simulink model "clearing_faulted_segment_travelling_Wave"  (R2018a)
settings: Solver=ode23t  StartTime=0.0  StopTime=2  MaxStep=1e-3  RelTol=1e-3
values from neighbouring files (symbols this model uses):
  AC_lim = [1.5 -1.5]    [MT_HVDC_initialize.m]
  C_pm = 10.48e-3    (= 0.01048)    [MT_HVDC_initialize.m]
  ccsc_lim = [1.0 -1.0]    [MT_HVDC_initialize.m]
  DC_lim = [1.05 -1.05]    [MT_HVDC_initialize.m]
  f = 50    [MT_HVDC_initialize.m]
  Fc = 50    [MT_HVDC_initialize.m]
  Fn_filter = 1000    [MT_HVDC_initialize.m]
  Ireg_lim_i = [1.5, -1.5]    [MT_HVDC_initialize.m]
  Ireg_lim_r = [1.5, -1.5]    [MT_HVDC_initialize.m]
  Ki_ACreg_i = 260    [MT_HVDC_initialize.m]
  Ki_ccsc = 5    [MT_HVDC_initialize.m]
  Ki_DCreg_r = 150    [MT_HVDC_initialize.m]
  Ki_Ireg_i = 200    [MT_HVDC_initialize.m]
  Ki_Ireg_r = 100    [MT_HVDC_initialize.m]
  Ki_R_inv = 150000    [MT_HVDC_initialize.m]
  Ki_R_rec = 5000    [MT_HVDC_initialize.m]
  Kp_ACreg_i = 2    [MT_HVDC_initialize.m]
  Kp_ccsc = 1    [MT_HVDC_initialize.m]
  Kp_DCreg_r = 8    [MT_HVDC_initialize.m]
  Kp_Ireg_i = 2    [MT_HVDC_initialize.m]
  Kp_Ireg_r = 2    [MT_HVDC_initialize.m]
  Kp_R_inv = 0.001    [MT_HVDC_initialize.m]
  Kp_R_rec = 0.001    [MT_HVDC_initialize.m]
  L1_pu = 0.109    [MT_HVDC_initialize.m]
  L2_pu = 0.0824    [MT_HVDC_initialize.m]
  L_arm = L_arm_pu*Z_base66/w    [MT_HVDC_initialize.m]
  L_arm_pu = 0.15    [MT_HVDC_initialize.m]
  L_int = X_int/w    [MT_HVDC_initialize.m]
  n = 50    [MT_HVDC_initialize.m]
  n2 = 50    [MT_HVDC_initialize.m]
  P_nom = 220e6    (= 220000000)    [MT_HVDC_initialize.m]
  R1_pu = 0.00206    [MT_HVDC_initialize.m]
  R2_pu = 0.00206    [MT_HVDC_initialize.m]
  R_arm = 0.03    [MT_HVDC_initialize.m]
  R_arm_pu = R_arm/Z_base66    [MT_HVDC_initialize.m]
  R_int = sqrt((z_int_400^2)/(1+xr_ratio^2))    [MT_HVDC_initialize.m]
  Rg_T1 = 40    [MT_HVDC_initialize.m]
  S1_nom = P_nom    (= 220000000)    [MT_HVDC_initialize.m]
  S2_nom = P_nom    (= 220000000)    [MT_HVDC_initialize.m]
  T_fault = 1.4    [MT_HVDC_initialize.m]
  Ts_Control = 40e-6    (= 4e-05)    [MT_HVDC_initialize.m]
  Ts_Power = 20e-6    (= 2e-05)    [MT_HVDC_initialize.m]
  V1_prim = V_prim    (= 400000)    [MT_HVDC_initialize.m]
  V1_sec = V_grid    (= 66000)    [MT_HVDC_initialize.m]
  V2_prim = V_grid    (= 66000)    [MT_HVDC_initialize.m]
  V2_sec = 18e3    (= 18000)    [MT_HVDC_initialize.m]
  V_ac_ref = 1.035    [MT_HVDC_initialize.m]
  V_grid = 66e3    (= 66000)    [MT_HVDC_initialize.m]
  V_prim = 400e3    (= 400000)    [MT_HVDC_initialize.m]
  Vc_pm_r = 0*Vdc_nom/n    (= 0)    [MT_HVDC_initialize.m]
  Vdc_nom = 135e3    (= 135000)    [MT_HVDC_initialize.m]
  w = 2*pi*f    (= 314.159265359)    [MT_HVDC_initialize.m]
  z0z1 = 0.8    [MT_HVDC_initialize.m]
  Zeta_filter = 1    [MT_HVDC_initialize.m]
undefined symbols (not defined in the file or in its folder): D1, Delta, DiscIntNeverNeededParam
libraries: powerlib x417, powerlib_meascontrol x130, simulink x84, powerlib_extras x8, simulink_extras x5
(part 2 of 17)

== system clearing_faulted_segment_travelling_Wave/Extra Sequences and functionality (Normally turned off) ==
  note: Iq controllers for converters
  note: Used for start-up simulation
  Enable Harmonic Filters : Step  Time=0  SampleTime=0
  Enable Reactive power setpoint regulation - (iq reference for inverter) : Step  Time=0.1  SampleTime=0
  Energize Converters with startup current - Bypasses startup resistors : Step  Time=0  SampleTime=0
  Energize grid Harmonic Filter : Step  Time=0.1  SampleTime=0
  Grid Voltage stabilizer TURN ON - (iq reference for rectifier) : Step  Time=999  SampleTime=0
  tag scope: T_Energize=global, T_Harmonic1=global, T_iq_reg_i=global, T_iq_reg_r=global, T_startup=global
  wires:
  Energize grid Harmonic Filter/1 -> [T_Energize]
  Enable Reactive power setpoint regulation - (iq reference for inverter)/1 -> [T_iq_reg_i]
  Energize Converters with startup current - Bypasses startup resistors/1 -> [T_startup]
  Grid Voltage stabilizer TURN ON - (iq reference for rectifier)/1 -> [T_iq_reg_r]
  Enable Harmonic Filters/1 -> [T_Harmonic1]

== system clearing_faulted_segment_travelling_Wave/GENERATOR 1 ==
  C1 : powerlib/Measurements/Three-Phase V-I Measurement  VoltageMeasurement=phase-to-ground  SetLabelV=on  LabelV=VC1  Vpu=off  VpuLL=off  CurrentMeasurement=yes  SetLabelI=on  LabelI=IC1  Ipu=off  Pbase=100e6  Vbase=500e3  OutputType=Complex  PhasorSimulation=off  PSBequivalent=0
      settings: SourceProductName=Simscape Electrical
  Grid Equivalent1 : powerlib/Elements/Three-Phase Mutual Inductance Z1-Z0  LConnTagsString=a|b|c  RConnTagsString=A|B|C  PositiveSequence="[ R  L]"  ZeroSequence="[ z0z1*L*w/7  z0z1*L]*0"
      settings: SourceProductName=Simscape Electrical  SourceProductBaseCode=PS
  Internal Source Impedance2 : powerlib/Elements/Three-Phase Series RLC Branch  Commented=on  LConnTagsString=A|B|C  RConnTagsString=A|B|C  BranchType=RL  Resistance=R  Inductance=L  Capacitance=1e-6  Measurements=None
      settings: SourceProductName=Simscape Electrical
  Phase A - Programmable : powerlib/Electrical Sources/Three-Phase Programmable Voltage Source  PositiveSequence="[V_g  0 F_s]"  VariationEntity=Amplitude  VariationType=Table of time-amplitude pairs  VariationTypeAlt=Step  VariationStep=-0.5  VariationRate=10  VariationMagnitude=0.3  VariationFrequency=2  VariationTiming=[6 6.15]  VariationPhaseA=off  Amplitudes=[1 (1+A) 1]  TimeValues=[0 T1 (T1+T2)]  HarmonicGeneration=off  HarmonicA=[3 0.2 -25 0]  HarmonicB=[2 0.15 35 2]  Timing="[0.05  3]"  BusType=swing  Pref=0  Qref=0  Qmin=-inf  Qmax=inf
      settings: SourceProductName=Simscape Electrical
  Phase B,C - Programmable : powerlib/Electrical Sources/Three-Phase Programmable Voltage Source  PositiveSequence="[V_g  0 f]"  VariationEntity=Amplitude  VariationType=Table of time-amplitude pairs  VariationTypeAlt=Step  VariationStep=-0.5  VariationRate=10  VariationMagnitude=0.3  VariationFrequency=2  VariationTiming=[6 6.15]  VariationPhaseA=off  Amplitudes=[1 (1+BC) 1]  TimeValues=[0 T1 (T1+T2)]  HarmonicGeneration=off  HarmonicA=[3 0.2 -25 0]  HarmonicB=[2 0.15 35 2]  Timing="[0.05  3]"  BusType=swing  Pref=50e6  Qref=50e6  Qmin=-inf  Qmax=inf
      settings: SourceProductName=Simscape Electrical
  A : PMIOPort  Side=Right
  B : PMIOPort  Port=2  Side=Right
  C : PMIOPort  Port=3  Side=Right
  N : PMIOPort  Tag=PMCPort  Port=4  Side=Left
  connections:
  Phase B,C - Programmable/LConn1 -- Phase A - Programmable/LConn1 -- N/RConn1
  Grid Equivalent1/LConn1 -- Phase A - Programmable/RConn1
  Grid Equivalent1/LConn2 -- Phase B,C - Programmable/RConn2
  Grid Equivalent1/LConn3 -- Phase B,C - Programmable/RConn3
  Grid Equivalent1/RConn3 -- C1/LConn3
  Grid Equivalent1/RConn2 -- C1/LConn2
  Grid Equivalent1/RConn1 -- C1/LConn1
  C1/RConn1 -- A/RConn1
  C1/RConn2 -- B/RConn1
  C1/RConn3 -- C/RConn1

== system clearing_faulted_segment_travelling_Wave/GENERATOR 2 ==
  C2 : powerlib/Measurements/Three-Phase V-I Measurement  VoltageMeasurement=phase-to-ground  SetLabelV=on  LabelV=VC2  Vpu=off  VpuLL=off  CurrentMeasurement=yes  SetLabelI=on  LabelI=IC2  Ipu=off  Pbase=100e6  Vbase=500e3  OutputType=Complex  PhasorSimulation=off  PSBequivalent=0
      settings: SourceProductName=Simscape Electrical
  Grid Equivalent1 : powerlib/Elements/Three-Phase Mutual Inductance Z1-Z0  LConnTagsString=a|b|c  RConnTagsString=A|B|C  PositiveSequence="[ R  L]"  ZeroSequence="[ z0z1*L*w/7  z0z1*L]*0"
      settings: SourceProductName=Simscape Electrical  SourceProductBaseCode=PS
  Internal Source Impedance2 : powerlib/Elements/Three-Phase Series RLC Branch  Commented=on  LConnTagsString=A|B|C  RConnTagsString=A|B|C  BranchType=RL  Resistance=R  Inductance=L  Capacitance=1e-6  Measurements=None
      settings: SourceProductName=Simscape Electrical
  Phase A - Programmable : powerlib/Electrical Sources/Three-Phase Programmable Voltage Source  PositiveSequence="[V_g  0 F_s]"  VariationEntity=Amplitude  VariationType=Table of time-amplitude pairs  VariationTypeAlt=Step  VariationStep=-0.5  VariationRate=10  VariationMagnitude=0.3  VariationFrequency=2  VariationTiming=[6 6.15]  VariationPhaseA=off  Amplitudes=[1 (1+A) 1]  TimeValues=[0 T1 (T1+T2)]  HarmonicGeneration=off  HarmonicA=[3 0.2 -25 0]  HarmonicB=[2 0.15 35 2]  Timing="[0.05  3]"  BusType=swing  Pref=0  Qref=0  Qmin=-inf  Qmax=inf
      settings: SourceProductName=Simscape Electrical
  Phase B,C - Programmable : powerlib/Electrical Sources/Three-Phase Programmable Voltage Source  PositiveSequence="[V_g  0 f]"  VariationEntity=Amplitude  VariationType=Table of time-amplitude pairs  VariationTypeAlt=Step  VariationStep=-0.5  VariationRate=10  VariationMagnitude=0.3  VariationFrequency=2  VariationTiming=[6 6.15]  VariationPhaseA=off  Amplitudes=[1 (1+BC) 1]  TimeValues=[0 T1 (T1+T2)]  HarmonicGeneration=off  HarmonicA=[3 0.2 -25 0]  HarmonicB=[2 0.15 35 2]  Timing="[0.05  3]"  BusType=swing  Pref=50e6  Qref=50e6  Qmin=-inf  Qmax=inf
      settings: SourceProductName=Simscape Electrical
  A : PMIOPort  Side=Right
  B : PMIOPort  Port=2  Side=Right
  C : PMIOPort  Port=3  Side=Right
  N : PMIOPort  Tag=PMCPort  Port=4  Side=Left
  connections:
  Phase B,C - Programmable/LConn1 -- Phase A - Programmable/LConn1 -- N/RConn1
  Grid Equivalent1/LConn1 -- Phase A - Programmable/RConn1
  Grid Equivalent1/LConn2 -- Phase B,C - Programmable/RConn2
  Grid Equivalent1/LConn3 -- Phase B,C - Programmable/RConn3
  Grid Equivalent1/RConn3 -- C2/LConn3
  Grid Equivalent1/RConn2 -- C2/LConn2
  Grid Equivalent1/RConn1 -- C2/LConn1
  C2/RConn1 -- A/RConn1
  C2/RConn2 -- B/RConn1
  C2/RConn3 -- C/RConn1

== system clearing_faulted_segment_travelling_Wave/GENERATOR 3 ==
  C3 : powerlib/Measurements/Three-Phase V-I Measurement  VoltageMeasurement=phase-to-ground  SetLabelV=on  LabelV=VC3  Vpu=off  VpuLL=off  CurrentMeasurement=yes  SetLabelI=on  LabelI=IC3  Ipu=off  Pbase=100e6  Vbase=500e3  OutputType=Complex  PhasorSimulation=off  PSBequivalent=0
      settings: SourceProductName=Simscape Electrical
  Grid Equivalent1 : powerlib/Elements/Three-Phase Mutual Inductance Z1-Z0  LConnTagsString=a|b|c  RConnTagsString=A|B|C  PositiveSequence="[ R  L]"  ZeroSequence="[ z0z1*L*w/7  z0z1*L]*0"
      settings: SourceProductName=Simscape Electrical  SourceProductBaseCode=PS
  Internal Source Impedance2 : powerlib/Elements/Three-Phase Series RLC Branch  Commented=on  LConnTagsString=A|B|C  RConnTagsString=A|B|C  BranchType=RL  Resistance=R  Inductance=L  Capacitance=1e-6  Measurements=None
      settings: SourceProductName=Simscape Electrical
  Phase A - Programmable : powerlib/Electrical Sources/Three-Phase Programmable Voltage Source  PositiveSequence="[V_g  0 F_s]"  VariationEntity=Amplitude  VariationType=Table of time-amplitude pairs  VariationTypeAlt=Step  VariationStep=-0.5  VariationRate=10  VariationMagnitude=0.3  VariationFrequency=2  VariationTiming=[6 6.15]  VariationPhaseA=off  Amplitudes=[1 (1+A) 1]  TimeValues=[0 T1 (T1+T2)]  HarmonicGeneration=off  HarmonicA=[3 0.2 -25 0]  HarmonicB=[2 0.15 35 2]  Timing="[0.05  3]"  BusType=swing  Pref=0  Qref=0  Qmin=-inf  Qmax=inf
      settings: SourceProductName=Simscape Electrical
  Phase B,C - Programmable : powerlib/Electrical Sources/Three-Phase Programmable Voltage Source  PositiveSequence="[V_g  0 f]"  VariationEntity=Amplitude  VariationType=Table of time-amplitude pairs  VariationTypeAlt=Step  VariationStep=-0.5  VariationRate=10  VariationMagnitude=0.3  VariationFrequency=2  VariationTiming=[6 6.15]  VariationPhaseA=off  Amplitudes=[1 (1+BC) 1]  TimeValues=[0 T1 (T1+T2)]  HarmonicGeneration=off  HarmonicA=[3 0.2 -25 0]  HarmonicB=[2 0.15 35 2]  Timing="[0.05  3]"  BusType=swing  Pref=50e6  Qref=50e6  Qmin=-inf  Qmax=inf
      settings: SourceProductName=Simscape Electrical
  A : PMIOPort  Side=Right
  B : PMIOPort  Port=2  Side=Right
  C : PMIOPort  Port=3  Side=Right
  N : PMIOPort  Tag=PMCPort  Port=4  Side=Left
  connections:
  Phase B,C - Programmable/LConn1 -- Phase A - Programmable/LConn1 -- N/RConn1
  Grid Equivalent1/LConn1 -- Phase A - Programmable/RConn1
  Grid Equivalent1/LConn2 -- Phase B,C - Programmable/RConn2
  Grid Equivalent1/LConn3 -- Phase B,C - Programmable/RConn3
  Grid Equivalent1/RConn3 -- C3/LConn3
  Grid Equivalent1/RConn2 -- C3/LConn2
  Grid Equivalent1/RConn1 -- C3/LConn1
  C3/RConn1 -- A/RConn1
  C3/RConn2 -- B/RConn1
  C3/RConn3 -- C/RConn1

== system clearing_faulted_segment_travelling_Wave/Harmonic Filters grid1 ==
  5 MVA - 3th : powerlib/Elements/Three-Phase Harmonic Filter  LConnTagsString=A|B|C  RConnTagsString=n  FilterType=Single-tuned  FilterConnection=Y (neutral)  ParNom=[V_grid f]  Qc=5e6  Fr=[3*f]  Frd=[11*60 13*60]  Q=100  Measurements=None
      settings: AttributesFormatString=\n  SourceProductName=Simscape Electrical  SourceProductBaseCode=PS
  5 MVA - HP : powerlib/Elements/Three-Phase Harmonic Filter  LConnTagsString=A|B|C  RConnTagsString=n  FilterType=High-pass  FilterConnection=Y (neutral)  ParNom=[V_grid f]  Qc=5e6  Fr=[33*f]  Frd=[11*60 13*60]  Q=100  Measurements=None
      settings: AttributesFormatString=\n  SourceProductName=Simscape Electrical  SourceProductBaseCode=PS
  Brk5 : powerlib/Elements/Three-Phase Breaker  InitialState=open  SwitchA=on  SwitchB=on  SwitchC=on  SwitchTimes=[30/60]*10000  External=on  BreakerResistance=0.001  SnubberResistance=1e6  SnubberCapacitance=inf  Measurements=None
      settings: SourceProductName=Simscape Electrical
  Ground4 : powerlib/Elements/Ground  LConnTagsString=a
      settings: SourceProductName=Simscape Electrical
  Three-Phase Series RLC Load : powerlib/Elements/Three-Phase Series RLC Load  LConnTagsString=A|B|C  Configuration=Y (grounded)  NominalVoltage=66e3  Vabc=[1e3 1e3 1e3]  Vabcp=[1e3 1e3 1e3]  NominalFrequency=f  UnbalancedPower=off  ActivePower=0  InductivePower=0  CapacitivePower=50e6  Pabc=[10e3 9e3 11e3]  QLabc=[100 90 110]  QCabc=[100 90 110]  Pabcp=[10e3 9e3 11e3]  QLabcp=[100 90 110]  QCabcp=[100 90 110]  Measurements=None  LoadType=constant Z
      settings: SourceProductName=Simscape Electrical
  A : PMIOPort  Tag=PMCPort  Side=Left
  B : PMIOPort  Tag=PMCPort  Port=2  Side=Left
  C : PMIOPort  Tag=PMCPort  Port=3  Side=Left
  wires:
  [T_Harmonic1] -> Brk5/1
  connections:
  Ground4/LConn1 -- 5 MVA - 3th/RConn1 -- 5 MVA - HP/RConn1
  5 MVA - 3th/LConn1 -- Three-Phase Series RLC Load/LConn1 -- Brk5/LConn1 -- 5 MVA - HP/LConn1
  5 MVA - 3th/LConn2 -- Three-Phase Series RLC Load/LConn2 -- Brk5/LConn2 -- 5 MVA - HP/LConn2
  5 MVA - 3th/LConn3 -- Three-Phase Series RLC Load/LConn3 -- Brk5/LConn3 -- 5 MVA - HP/LConn3
  Brk5/RConn1 -- A/RConn1
  Brk5/RConn2 -- B/RConn1
  Brk5/RConn3 -- C/RConn1

== system clearing_faulted_segment_travelling_Wave/Harmonic Filters grid2 ==
  10 MVA - 3 & 5th : powerlib/Elements/Three-Phase Harmonic Filter  LConnTagsString=A|B|C  RConnTagsString=n  FilterType=Double-tuned  FilterConnection=Y (neutral)  ParNom=[V_grid f]  Qc=5e6  Fr=[3*f]  Frd=[5*f 7*f]  Q=100  Measurements=None
      settings: AttributesFormatString=\n  SourceProductName=Simscape Electrical  SourceProductBaseCode=PS
  10 MVA - 3 & 5th1 : powerlib/Elements/Three-Phase Harmonic Filter  LConnTagsString=A|B|C  RConnTagsString=n  FilterType=Single-tuned  FilterConnection=Y (neutral)  ParNom=[V_grid f]  Qc=2e6  Fr=[13*f]  Frd=[5*f 7*f]  Q=100  Measurements=None
      settings: AttributesFormatString=\n  SourceProductName=Simscape Electrical  SourceProductBaseCode=PS
  5 MVA - 7th : powerlib/Elements/Three-Phase Harmonic Filter  LConnTagsString=A|B|C  RConnTagsString=n  FilterType=Double-tuned  FilterConnection=Y (neutral)  ParNom=[V_grid f]  Qc=3e6  Fr=[40*f]  Frd=[9*f 11*f]  Q=100  Measurements=None
      settings: AttributesFormatString=\n  SourceProductName=Simscape Electrical  SourceProductBaseCode=PS
  Brk5 : powerlib/Elements/Three-Phase Breaker  InitialState=open  SwitchA=on  SwitchB=on  SwitchC=on  SwitchTimes=[30/60]*10000  External=on  BreakerResistance=0.001  SnubberResistance=1e6  SnubberCapacitance=inf  Measurements=None
      settings: SourceProductName=Simscape Electrical
  Ground4 : powerlib/Elements/Ground  Commented=on  LConnTagsString=a
      settings: SourceProductName=Simscape Electrical
  HP 21th : powerlib/Elements/Three-Phase Harmonic Filter  LConnTagsString=A|B|C  RConnTagsString=n  FilterType=High-pass  FilterConnection=Y (neutral)  ParNom=[V_grid f]  Qc=3e6  Fr=[21*f]  Frd=[11*60 13*60]  Q=100  Measurements=None
      settings: AttributesFormatString=\n  SourceProductName=Simscape Electrical  SourceProductBaseCode=PS
  HP 35th : powerlib/Elements/Three-Phase Harmonic Filter  LConnTagsString=A|B|C  RConnTagsString=n  FilterType=High-pass  FilterConnection=Y (neutral)  ParNom=[V_grid f]  Qc=3e6  Fr=[35*f]  Frd=[11*60 13*60]  Q=100  Measurements=None
      settings: AttributesFormatString=\n  SourceProductName=Simscape Electrical  SourceProductBaseCode=PS
  A : PMIOPort  Tag=PMCPort  Side=Left
  B : PMIOPort  Tag=PMCPort  Port=2  Side=Left
  C : PMIOPort  Tag=PMCPort  Port=3  Side=Left
  wires:
  [T_Harmonic1] -> Brk5/1
  connections:
  HP 35th/LConn3 -- Brk5/LConn3 -- 10 MVA - 3 & 5th1/LConn3 -- HP 21th/LConn3 -- 10 MVA - 3 & 5th/LConn3 -- 5 MVA - 7th/LConn3
  HP 35th/LConn2 -- Brk5/LConn2 -- 10 MVA - 3 & 5th1/LConn2 -- HP 21th/LConn2 -- 10 MVA - 3 & 5th/LConn2 -- 5 MVA - 7th/LConn2
  HP 35th/LConn1 -- HP 21th/LConn1 -- 10 MVA - 3 & 5th1/LConn1 -- 10 MVA - 3 & 5th/LConn1 -- 5 MVA - 7th/LConn1 -- Brk5/LConn1
  5 MVA - 7th/RConn1 -- Ground4/LConn1 -- HP 35th/RConn1 -- 10 MVA - 3 & 5th1/RConn1 -- HP 21th/RConn1 -- 10 MVA - 3 & 5th/RConn1
  Brk5/RConn1 -- A/RConn1
  B/RConn1 -- Brk5/RConn2
  Brk5/RConn3 -- C/RConn1

== system clearing_faulted_segment_travelling_Wave/Harmonic Filters grid3 ==
  10 MVA - 3 & 5th : powerlib/Elements/Three-Phase Harmonic Filter  LConnTagsString=A|B|C  RConnTagsString=n  FilterType=Double-tuned  FilterConnection=Y (neutral)  ParNom=[V_grid f]  Qc=5e6  Fr=[3*f]  Frd=[5*f 7*f]  Q=100  Measurements=None
      settings: AttributesFormatString=\n  SourceProductName=Simscape Electrical  SourceProductBaseCode=PS
  10 MVA - 3 & 5th1 : powerlib/Elements/Three-Phase Harmonic Filter  LConnTagsString=A|B|C  RConnTagsString=n  FilterType=Single-tuned  FilterConnection=Y (neutral)  ParNom=[V_grid f]  Qc=2e6  Fr=[13*f]  Frd=[5*f 7*f]  Q=100  Measurements=None
      settings: AttributesFormatString=\n  SourceProductName=Simscape Electrical  SourceProductBaseCode=PS
  5 MVA - 7th : powerlib/Elements/Three-Phase Harmonic Filter  LConnTagsString=A|B|C  RConnTagsString=n  FilterType=Double-tuned  FilterConnection=Y (neutral)  ParNom=[V_grid f]  Qc=3e6  Fr=[40*f]  Frd=[9*f 11*f]  Q=100  Measurements=None
      settings: AttributesFormatString=\n  SourceProductName=Simscape Electrical  SourceProductBaseCode=PS
  Brk5 : powerlib/Elements/Three-Phase Breaker  InitialState=open  SwitchA=on  SwitchB=on  SwitchC=on  SwitchTimes=[30/60]*10000  External=on  BreakerResistance=0.001  SnubberResistance=1e6  SnubberCapacitance=inf  Measurements=None
      settings: SourceProductName=Simscape Electrical
  Ground4 : powerlib/Elements/Ground  Commented=on  LConnTagsString=a
      settings: SourceProductName=Simscape Electrical
  HP 21th : powerlib/Elements/Three-Phase Harmonic Filter  LConnTagsString=A|B|C  RConnTagsString=n  FilterType=High-pass  FilterConnection=Y (neutral)  ParNom=[V_grid f]  Qc=3e6  Fr=[21*f]  Frd=[11*60 13*60]  Q=100  Measurements=None
      settings: AttributesFormatString=\n  SourceProductName=Simscape Electrical  SourceProductBaseCode=PS
  HP 35th : powerlib/Elements/Three-Phase Harmonic Filter  LConnTagsString=A|B|C  RConnTagsString=n  FilterType=High-pass  FilterConnection=Y (neutral)  ParNom=[V_grid f]  Qc=3e6  Fr=[35*f]  Frd=[11*60 13*60]  Q=100  Measurements=None
      settings: AttributesFormatString=\n  SourceProductName=Simscape Electrical  SourceProductBaseCode=PS
  A : PMIOPort  Tag=PMCPort  Side=Left
  B : PMIOPort  Tag=PMCPort  Port=2  Side=Left
  C : PMIOPort  Tag=PMCPort  Port=3  Side=Left
  wires:
  [T_Harmonic1] -> Brk5/1
  connections:
  HP 35th/LConn3 -- Brk5/LConn3 -- 10 MVA - 3 & 5th1/LConn3 -- HP 21th/LConn3 -- 10 MVA - 3 & 5th/LConn3 -- 5 MVA - 7th/LConn3
  HP 35th/LConn2 -- Brk5/LConn2 -- 10 MVA - 3 & 5th1/LConn2 -- HP 21th/LConn2 -- 10 MVA - 3 & 5th/LConn2 -- 5 MVA - 7th/LConn2
  HP 35th/LConn1 -- HP 21th/LConn1 -- 10 MVA - 3 & 5th1/LConn1 -- 10 MVA - 3 & 5th/LConn1 -- 5 MVA - 7th/LConn1 -- Brk5/LConn1
  5 MVA - 7th/RConn1 -- Ground4/LConn1 -- HP 35th/RConn1 -- 10 MVA - 3 & 5th1/RConn1 -- HP 21th/RConn1 -- 10 MVA - 3 & 5th/RConn1
  Brk5/RConn1 -- A/RConn1
  B/RConn1 -- Brk5/RConn2
  Brk5/RConn3 -- C/RConn1

== system clearing_faulted_segment_travelling_Wave/Harmonic Filters grid4 ==
  10 MVA - 3 & 5th : powerlib/Elements/Three-Phase Harmonic Filter  LConnTagsString=A|B|C  RConnTagsString=n  FilterType=Double-tuned  FilterConnection=Y (neutral)  ParNom=[V_grid f]  Qc=5e6  Fr=[3*f]  Frd=[5*f 7*f]  Q=100  Measurements=None
      settings: AttributesFormatString=\n  SourceProductName=Simscape Electrical  SourceProductBaseCode=PS
  10 MVA - 3 & 5th1 : powerlib/Elements/Three-Phase Harmonic Filter  LConnTagsString=A|B|C  RConnTagsString=n  FilterType=Single-tuned  FilterConnection=Y (neutral)  ParNom=[V_grid f]  Qc=2e6  Fr=[13*f]  Frd=[5*f 7*f]  Q=100  Measurements=None
      settings: AttributesFormatString=\n  SourceProductName=Simscape Electrical  SourceProductBaseCode=PS
  5 MVA - 7th : powerlib/Elements/Three-Phase Harmonic Filter  LConnTagsString=A|B|C  RConnTagsString=n  FilterType=Double-tuned  FilterConnection=Y (neutral)  ParNom=[V_grid f]  Qc=3e6  Fr=[40*f]  Frd=[9*f 11*f]  Q=100  Measurements=None
      settings: AttributesFormatString=\n  SourceProductName=Simscape Electrical  SourceProductBaseCode=PS
  Brk5 : powerlib/Elements/Three-Phase Breaker  InitialState=open  SwitchA=on  SwitchB=on  SwitchC=on  SwitchTimes=[30/60]*10000  External=on  BreakerResistance=0.001  SnubberResistance=1e6  SnubberCapacitance=inf  Measurements=None
      settings: SourceProductName=Simscape Electrical
  Ground4 : powerlib/Elements/Ground  Commented=on  LConnTagsString=a
      settings: SourceProductName=Simscape Electrical
  HP 21th : powerlib/Elements/Three-Phase Harmonic Filter  LConnTagsString=A|B|C  RConnTagsString=n  FilterType=High-pass  FilterConnection=Y (neutral)  ParNom=[V_grid f]  Qc=3e6  Fr=[21*f]  Frd=[11*60 13*60]  Q=100  Measurements=None
      settings: AttributesFormatString=\n  SourceProductName=Simscape Electrical  SourceProductBaseCode=PS
  HP 35th : powerlib/Elements/Three-Phase Harmonic Filter  LConnTagsString=A|B|C  RConnTagsString=n  FilterType=High-pass  FilterConnection=Y (neutral)  ParNom=[V_grid f]  Qc=3e6  Fr=[35*f]  Frd=[11*60 13*60]  Q=100  Measurements=None
      settings: AttributesFormatString=\n  SourceProductName=Simscape Electrical  SourceProductBaseCode=PS
  A : PMIOPort  Tag=PMCPort  Side=Left
  B : PMIOPort  Tag=PMCPort  Port=2  Side=Left
  C : PMIOPort  Tag=PMCPort  Port=3  Side=Left
  wires:
  [T_Harmonic1] -> Brk5/1
  connections:
  HP 35th/LConn3 -- Brk5/LConn3 -- 10 MVA - 3 & 5th1/LConn3 -- HP 21th/LConn3 -- 10 MVA - 3 & 5th/LConn3 -- 5 MVA - 7th/LConn3
  HP 35th/LConn2 -- Brk5/LConn2 -- 10 MVA - 3 & 5th1/LConn2 -- HP 21th/LConn2 -- 10 MVA - 3 & 5th/LConn2 -- 5 MVA - 7th/LConn2
  HP 35th/LConn1 -- HP 21th/LConn1 -- 10 MVA - 3 & 5th1/LConn1 -- 10 MVA - 3 & 5th/LConn1 -- 5 MVA - 7th/LConn1 -- Brk5/LConn1
  5 MVA - 7th/RConn1 -- Ground4/LConn1 -- HP 35th/RConn1 -- 10 MVA - 3 & 5th1/RConn1 -- HP 21th/RConn1 -- 10 MVA - 3 & 5th/RConn1
  Brk5/RConn1 -- A/RConn1
  B/RConn1 -- Brk5/RConn2
  Brk5/RConn3 -- C/RConn1

== system clearing_faulted_segment_travelling_Wave/Load System ==
  200 MVA : powerlib/Elements/Three-Phase Series RLC Load  LConnTagsString=A|B|C  Configuration=Y (grounded)  NominalVoltage=18e3  Vabc=[1e3 1e3 1e3]  Vabcp=[1e3 1e3 1e3]  NominalFrequency=f  UnbalancedPower=off  ActivePower=P_load  InductivePower=Q_load  CapacitivePower=0  Pabc=[10e3 9e3 11e3]  QLabc=[100 90 110]  QCabc=[100 90 110]  Pabcp=[10e3 9e3 11e3]  QLabcp=[100 90 110]  QCabcp=[100 90 110]  Measurements=None  LoadType=constant PQ
      settings: SourceProductName=Simscape Electrical
  Brk1 : powerlib/Elements/Three-Phase Breaker  InitialState=open  SwitchA=on  SwitchB=on  SwitchC=on  SwitchTimes=[30/60]*10000  External=on  BreakerResistance=0.01  SnubberResistance=1e6  SnubberCapacitance=inf  Measurements=None
      settings: SourceProductName=Simscape Electrical
  Nominal Load1 : powerlib/Measurements/Three-Phase V-I Measurement  VoltageMeasurement=phase-to-ground  SetLabelV=on  LabelV=Vabc_load  Vpu=off  VpuLL=off  CurrentMeasurement=yes  SetLabelI=on  LabelI=Iabc_load  Ipu=off  Pbase=100e6  Vbase=18e3  OutputType=Magnitude  PhasorSimulation=off  PSBequivalent=0
      settings: SourceProductName=Simscape Electrical
  A : PMIOPort  Side=Left
  B : PMIOPort  Port=2  Side=Left
  C : PMIOPort  Port=3  Side=Left
  wires:
  [T_Load_nom] -> Brk1/1
  connections:
  Nominal Load1/RConn3 -- 200 MVA/LConn1
  Nominal Load1/RConn2 -- 200 MVA/LConn2
  Nominal Load1/RConn1 -- 200 MVA/LConn3
  A/RConn1 -- Brk1/LConn1
  B/RConn1 -- Brk1/LConn2
  C/RConn1 -- Brk1/LConn3
  Brk1/RConn3 -- Nominal Load1/LConn1
  Brk1/RConn2 -- Nominal Load1/LConn2
  Brk1/RConn1 -- Nominal Load1/LConn3
